simulink model "MDriverRegenRequested"  (R2024b)
settings: Solver=FixedStepAuto  StartTime=0.0  StopTime=10.0  RelTol=1e-3  EnableMultiTasking=on
undefined symbols (not defined in the file): IRegen15C, IRegen6C, MNominal, rGearboxRatio, rTyreRadius, tMaxRegen, tTorqueControlTask
libraries: simulink x5
settings Model: DataDictionary=Master_Dictionary.sldd  EnableAccessToBaseWorkspace=off  Creator=torni  LastModifiedBy=Will
settings OptimizationCC: DefaultParameterBehavior=Inlined  EnhancedBackFolding=on  PassReuseOutputArgsAs=Individual arguments  ZeroExternalMemoryAtStartup=off  ZeroInternalMemoryAtStartup=off  MaxStackSize=8192  OptimizeBlockOrder=speed  DifferentSizesBufferReuse=on  OptimizationCustomize=off  EfficientTunableParamExpr=on
settings DebuggingCC: ParameterTunabilityLossMsg=error
settings HardwareCC: ProdBitPerPointer=32  ProdBitPerSizeT=32  ProdBitPerPtrDiffT=32  ProdLargestAtomicInteger=Long  ProdLargestAtomicFloat=Double  ProdWordSize=32  ProdLongLongMode=on  ProdHWDeviceType=ARM Compatible->ARM Cortex-M
settings SFSimCC: MATLABDynamicMemAlloc=off
settings RTWCC: Description=Embedded Coder  SystemTargetFile=ert.tlc  HardwareBoard=STM32H7xx Based (Single-core)  TemplateMakefile=ert_default_tmf  Toolchain=GNU Tools for ARM Embedded Processors
settings CodeAppCC: ForceParamTrailComments=on  IgnoreCustomStorageClasses=off  OperatorAnnotations=on  SimulinkDataObjDesc=on  SFDataObjDesc=on  InsertBlockDesc=on
settings ERTTargetCC: TargetLangStandard=C99 (ISO)  CodeReplacementLibrary=ARM Cortex-M  ExtModeTransport=3  ExtModeStaticAlloc=on  ExtModeStaticAllocSize=2048  ExtModeMexFile=ext_xcp  ExtModeIntrfLevel=Level2 - Open

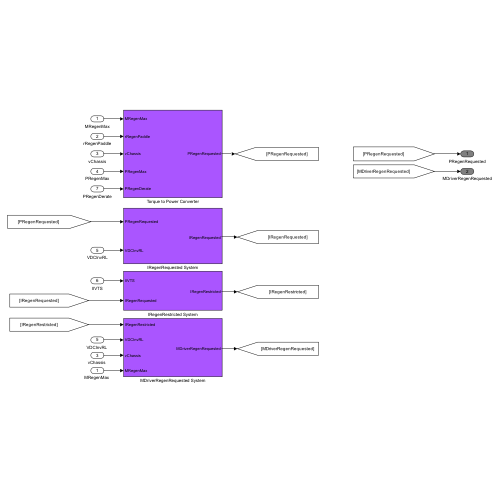
[thumbnail: Simulink's stored preview of the top-level diagram]
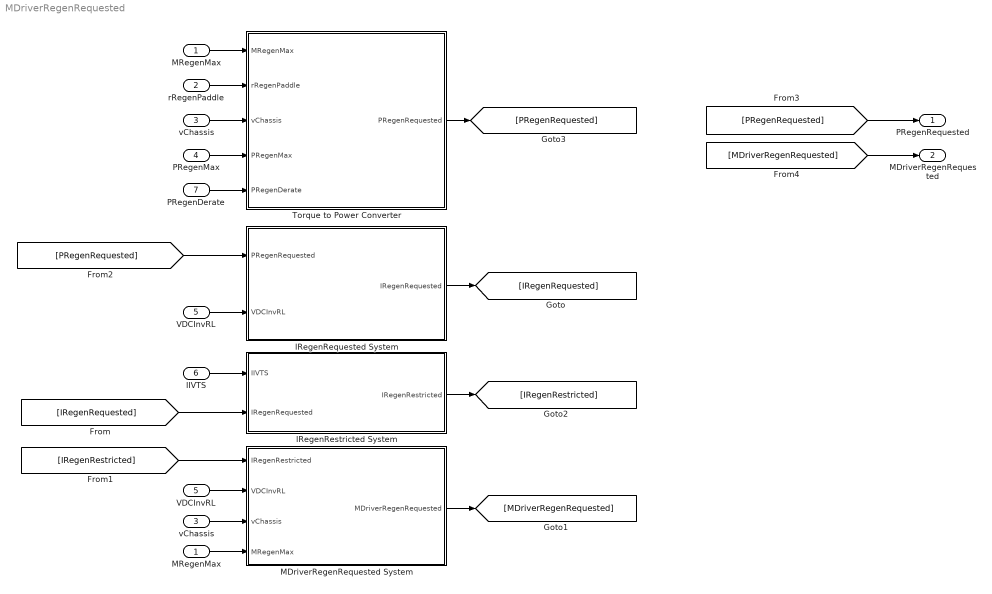
== system MDriverRegenRequested ==
  MRegenMax : Inport  OutDataTypeStr=double
  rRegenPaddle : Inport  Port=2  OutDataTypeStr=double
  vChassis : Inport  Port=3  OutDataTypeStr=double
  PRegenMax : Inport  Port=4  OutDataTypeStr=double
  VDCInvRL : Inport  Port=5  OutDataTypeStr=double
  IIVTS : Inport  Port=6  OutDataTypeStr=double
  PRegenDerate : Inport  Port=7  OutDataTypeStr=double
  IRegenRequested System : Subsystem
  IRegenRestricted System : Subsystem
  "MDriverRegenRequested System " : Subsystem
  "MRegenMax " : InportShadow  OutDataTypeStr=double
  Torque to Power Converter : Subsystem
  "VDCInvRL " : InportShadow  Port=5  OutDataTypeStr=double
  "vChassis " : InportShadow  Port=3  OutDataTypeStr=double
  PRegenRequested : Outport  OutDataTypeStr=double  VectorParamsAs1DForOutWhenUnconnected=off
  MDriverRegenRequested : Outport  Port=2  OutDataTypeStr=double  VectorParamsAs1DForOutWhenUnconnected=off
  wires:
  vChassis/1 -> Torque to Power Converter/3(vChassis)
  IRegenRequested System/1(IRegenRequested) -> [IRegenRequested]
  "vChassis "/1 -> "MDriverRegenRequested System "/3(vChassis)
  [IRegenRequested] -> IRegenRestricted System/2(IRegenRequested)
  Torque to Power Converter/1(PRegenRequested) -> [PRegenRequested]
  [IRegenRestricted] -> "MDriverRegenRequested System "/1(IRegenRestricted)
  rRegenPaddle/1 -> Torque to Power Converter/2(rRegenPaddle)
  "VDCInvRL "/1 -> "MDriverRegenRequested System "/2(VDCInvRL)
  IRegenRestricted System/1(IRegenRestricted) -> [IRegenRestricted]
  IIVTS/1 -> IRegenRestricted System/1(IIVTS)
  PRegenMax/1 -> Torque to Power Converter/4(PRegenMax)
  MRegenMax/1 -> Torque to Power Converter/1(MRegenMax)
  VDCInvRL/1 -> IRegenRequested System/2(VDCInvRL)
  [PRegenRequested] -> IRegenRequested System/1(PRegenRequested)
  [PRegenRequested] -> PRegenRequested/1
  "MDriverRegenRequested System "/1(MDriverRegenRequested) -> [MDriverRegenRequested]
  [MDriverRegenRequested] -> MDriverRegenRequested/1
  "MRegenMax "/1 -> "MDriverRegenRequested System "/4(MRegenMax)
  PRegenDerate/1 -> Torque to Power Converter/5(PRegenDerate)

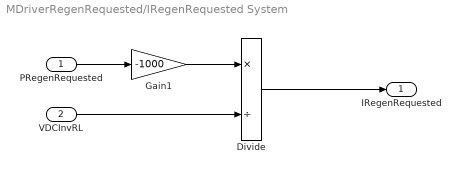
== system MDriverRegenRequested/IRegenRequested System ==
  PRegenRequested : Inport  OutDataTypeStr=double
  VDCInvRL : Inport  Port=2  OutDataTypeStr=double
  Divide : Product  Inputs=*/
  Gain1 : Gain  Gain=-1000
  IRegenRequested : Outport  OutDataTypeStr=double  VectorParamsAs1DForOutWhenUnconnected=off
  wires:
  Divide/1 -> IRegenRequested/1
  VDCInvRL/1 -> Divide/2
  PRegenRequested/1 -> Gain1/1
  Gain1/1 -> Divide/1

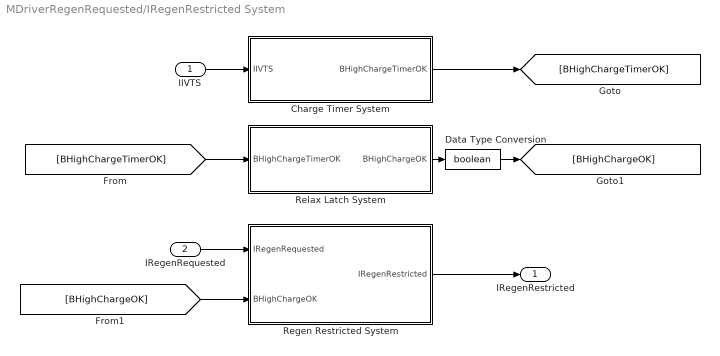
== system MDriverRegenRequested/IRegenRestricted System ==
  IIVTS : Inport  OutDataTypeStr=double
  IRegenRequested : Inport  Port=2  OutDataTypeStr=double
  Charge Timer System : Subsystem
  Data Type Conversion : DataTypeConversion  OutDataTypeStr=boolean  SaturateOnIntegerOverflow=off  RndMeth=Floor
  Regen Restricted System : Subsystem
  Relax Latch System : Stateflow chart  TreatAsAtomicUnit=on
  IRegenRestricted : Outport  OutDataTypeStr=double  VectorParamsAs1DForOutWhenUnconnected=off
  wires:
  IIVTS/1 -> Charge Timer System/1(IIVTS)
  Charge Timer System/1(BHighChargeTimerOK) -> [BHighChargeTimerOK]
  [BHighChargeTimerOK] -> Relax Latch System/1(BHighChargeTimerOK)
  IRegenRequested/1 -> Regen Restricted System/1(IRegenRequested)
  [BHighChargeOK] -> Regen Restricted System/2(BHighChargeOK)
  Regen Restricted System/1(IRegenRestricted) -> IRegenRestricted/1
  Relax Latch System/1(BHighChargeOK) -> Data Type Conversion/1
  Data Type Conversion/1 -> [BHighChargeOK]

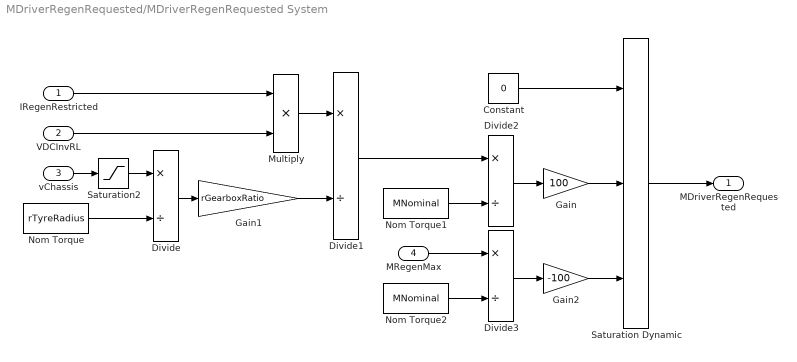
== system MDriverRegenRequested/MDriverRegenRequested System  ==
  IRegenRestricted : Inport
  VDCInvRL : Inport  Port=2
  vChassis : Inport  Port=3
  MRegenMax : Inport  Port=4
  Constant : Constant  Value=0
  Divide{,1..3} (4 alike) : Product  Inputs=*/
  Gain : Gain  Gain=100
  Gain1 : Gain  Gain=rGearboxRatio
  Gain2 : Gain  Gain=-100
  Multiply : Product
  Nom Torque : Constant  Value=rTyreRadius
  Nom Torque1 : Constant  Value=MNominal
  Nom Torque2 : Constant  Value=MNominal
  Saturation Dynamic : simulink/Discontinuities/Saturation Dynamic  OutMin=[]  OutMax=[]  OutDataTypeStr=Inherit: Same as second input  OutDataType=fixdt(1, 16)  OutScaling=2^-10  DoSatur=off
  Saturation2 : Saturate  UpperLimit=40  LowerLimit=0.1
  MDriverRegenRequested : Outport  VectorParamsAs1DForOutWhenUnconnected=off
  wires:
  Gain/1 -> Saturation Dynamic/2
  Saturation Dynamic/1 -> MDriverRegenRequested/1
  VDCInvRL/1 -> Multiply/2
  IRegenRestricted/1 -> Multiply/1
  Nom Torque/1 -> Divide/2
  Multiply/1 -> Divide1/1
  Divide/1 -> Gain1/1
  Divide1/1 -> Divide2/1
  Divide2/1 -> Gain/1
  Nom Torque1/1 -> Divide2/2
  vChassis/1 -> Saturation2/1
  Gain1/1 -> Divide1/2
  Nom Torque2/1 -> Divide3/2
  Divide3/1 -> Gain2/1
  MRegenMax/1 -> Divide3/1
  Gain2/1 -> Saturation Dynamic/3
  Constant/1 -> Saturation Dynamic/1
  Saturation2/1 -> Divide/1

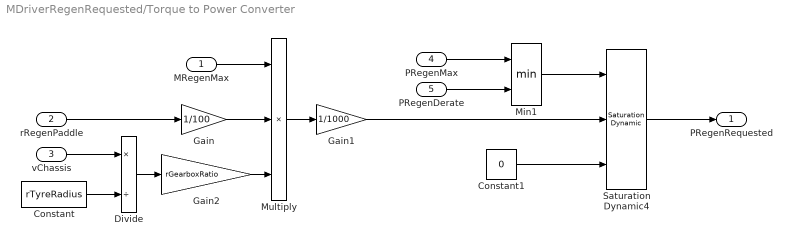
== system MDriverRegenRequested/Torque to Power Converter ==
  MRegenMax : Inport  OutDataTypeStr=double
  rRegenPaddle : Inport  Port=2  OutDataTypeStr=double
  vChassis : Inport  Port=3  OutDataTypeStr=double
  PRegenMax : Inport  Port=4
  PRegenDerate : Inport  Port=5
  Constant : Constant  Value=rTyreRadius  SampleTime=-1
  Constant1 : Constant  Value=0
  Divide : Product  Inputs=*/
  Gain : Gain  Gain=1/100
  Gain1 : Gain  Gain=1/1000
  Gain2 : Gain  Gain=rGearboxRatio
  Min1 : MinMax  Inputs=2
  Multiply : Product  Inputs=3
  Saturation Dynamic4 : simulink/Discontinuities/Saturation Dynamic  OutMin=[]  OutMax=[]  OutDataTypeStr=double  OutputDataTypeScalingMode=double  OutDataType=fixdt(1, 16)  OutScaling=2^-10  DoSatur=off
  PRegenRequested : Outport  OutDataTypeStr=double  VectorParamsAs1DForOutWhenUnconnected=off
  wires:
  Gain/1 -> Multiply/2
  rRegenPaddle/1 -> Gain/1
  vChassis/1 -> Divide/1
  Multiply/1 -> Gain1/1
  Saturation Dynamic4/1 -> PRegenRequested/1
  Divide/1 -> Gain2/1
  Constant/1 -> Divide/2
  Constant1/1 -> Saturation Dynamic4/3
  Gain1/1 -> Saturation Dynamic4/2
  MRegenMax/1 -> Multiply/1
  Gain2/1 -> Multiply/3
  Min1/1 -> Saturation Dynamic4/1
  PRegenDerate/1 -> Min1/2
  PRegenMax/1 -> Min1/1

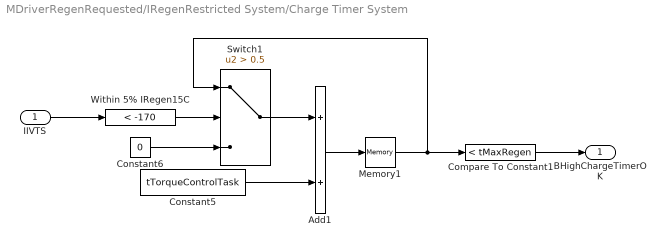
== system MDriverRegenRequested/IRegenRestricted System/Charge Timer System ==
  IIVTS : Inport  OutDataTypeStr=double
  Add1 : Sum
  Compare To Constant1 : simulink/Logic and Bit Operations/Compare To Constant  relop=<  const=tMaxRegen  OutDataTypeStr=boolean
  Constant5 : Constant  Value=tTorqueControlTask
  Constant6 : Constant  Value=0
  Memory1 : Memory  InheritSampleTime=on
  Switch1 : Switch  Criteria=u2 > Threshold  Threshold=0.5  SaturateOnIntegerOverflow=off  InputSameDT=off
  Within 5% IRegen15C : simulink/Logic and Bit Operations/Compare To Constant  relop=<  const=-170  OutDataTypeStr=boolean
  BHighChargeTimerOK : Outport  OutDataTypeStr=boolean  VectorParamsAs1DForOutWhenUnconnected=off
  wires:
  Compare To Constant1/1 -> BHighChargeTimerOK/1
  Memory1/1 -> Compare To Constant1/1, Switch1/1
  Switch1/1 -> Add1/1
  Add1/1 -> Memory1/1
  Within 5% IRegen15C/1 -> Switch1/2
  Constant5/1 -> Add1/2
  Constant6/1 -> Switch1/3
  IIVTS/1 -> Within 5% IRegen15C/1

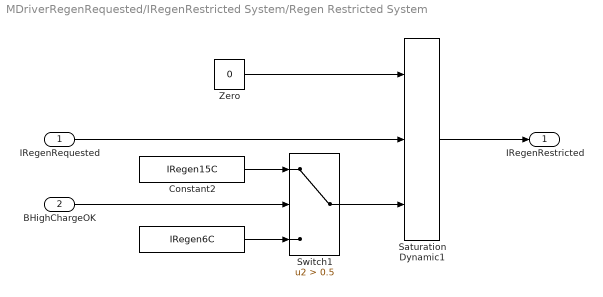
== system MDriverRegenRequested/IRegenRestricted System/Regen Restricted System ==
  IRegenRequested : Inport  OutDataTypeStr=double
  BHighChargeOK : Inport  Port=2  OutDataTypeStr=boolean
  " " : Constant  Value=IRegen6C
  Constant2 : Constant  Value=IRegen15C
  Saturation Dynamic1 : simulink/Discontinuities/Saturation Dynamic  OutMin=[]  OutMax=[]  OutDataTypeStr=Inherit: Same as second input  OutDataType=fixdt(1, 16)  OutScaling=2^-10  DoSatur=off
  Switch1 : Switch  Criteria=u2 > Threshold  Threshold=0.5  SaturateOnIntegerOverflow=off  InputSameDT=off
  Zero : Constant  Value=0  SampleTime=-1
  IRegenRestricted : Outport  OutDataTypeStr=double  VectorParamsAs1DForOutWhenUnconnected=off
  wires:
  Saturation Dynamic1/1 -> IRegenRestricted/1
  Switch1/1 -> Saturation Dynamic1/3
  IRegenRequested/1 -> Saturation Dynamic1/2
  " "/1 -> Switch1/3
  Constant2/1 -> Switch1/1
  Zero/1 -> Saturation Dynamic1/1
  BHighChargeOK/1 -> Switch1/2

== stateflow chart MDriverRegenRequested/IRegenRestricted System/Relax Latch System ==
  state Reset
    BHighChargeOK = 0;
  state Entrance
    entry:
    BHighChargeOK = 1;
  Entrance -> Reset : [BHighChargeTimerOK<0.5]
  (default) -> Entrance
  Reset -> Entrance : after(5000,tick)
  data: BHighChargeTimerOK input boolean; BHighChargeOK output double
